simulink model "Maxpid_correction_veleves"  (R2015b)
settings: Solver=ode45  StartTime=0.0  StopTime=1  MaxStep=0.01  RelTol=1e-3
undefined symbols (not defined in the file): Cext, Kd, Ki, Kp
settings Model: Creator=antomart  LastModifiedBy=David
settings DataIOCC: LimitDataPoints=off  SaveFormat=StructureWithTime
settings HardwareCC: ProdWordSize=32  ProdHWDeviceType=Specified
settings ModelReferenceCC: PropagateSignalLabelsOutOfModel=on
settings GRTTargetCC: GeneratePreprocessorConditionals=Disable all

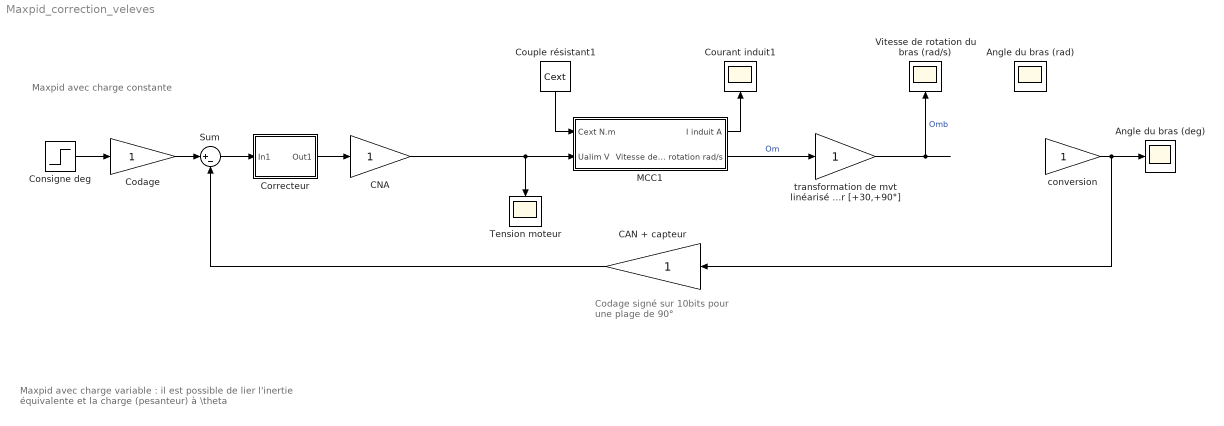
== system Maxpid_correction_veleves ==
  note: Maxpid avec charge variable : il est possible de lier l'inertie équivalente et la charge (pesanteur) à \theta
  note: Maxpid avec charge constante
  note: Codage signé sur 10bits pour une plage de 90°
  Angle du bras (rad) : Scope
  Angle du bras (deg) : Scope
  CAN + capteur : Gain
  CNA : Gain
  Codage : Gain
  Consigne deg : Step  Time=0  After=30  SampleTime=0
  Correcteur : Subsystem
  Couple résistant1 : Constant  Value=Cext
  Courant induit1 : Scope
  MCC1 : Subsystem
  Sum : Sum  Inputs=|+-
  Tension moteur : Scope
  Vitesse de rotation du bras (rad/s) : Scope
  conversion : Gain
  transformation de mvt linéarisé sur [+30,+90°] : Gain
  wires:
  Couple résistant1/1 -> MCC1/1(Cext N.m)
  MCC1/1(I induit A) -> Courant induit1/1
  MCC1/2(Vitesse de rotation rad/s) -> transformation de mvt linéarisé sur [+30,+90°]/1  "Om"
  transformation de mvt linéarisé sur [+30,+90°]/1 -> Vitesse de rotation du bras (rad/s)/1  "Omb"
  ? -> conversion/1, Angle du bras (rad)/1  "Thb (rad)"
  Sum/1 -> Correcteur/1(In1)
  Correcteur/1(Out1) -> CNA/1
  Consigne deg/1 -> Codage/1
  CAN + capteur/1 -> Sum/2
  Codage/1 -> Sum/1
  conversion/1 -> CAN + capteur/1, Angle du bras (deg)/1
  CNA/1 -> MCC1/2(Ualim V), Tension moteur/1

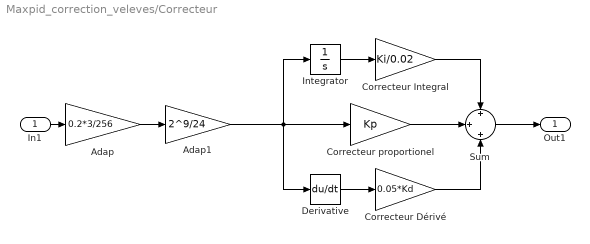
== system Maxpid_correction_veleves/Correcteur ==
  In1 : Inport
  Adap : Gain  Gain=0.2*3/256
  Adap1 : Gain  Gain=2^9/24
  Correcteur Dérivé : Gain  Gain=0.05*Kd
  Correcteur Integral : Gain  Gain=Ki/0.02
  Correcteur proportionel : Gain  Gain=Kp
  Derivative : Derivative
  Integrator : Integrator
  Sum : Sum  Inputs=+|+|+
  Out1 : Outport
  wires:
  In1/1 -> Adap/1
  Integrator/1 -> Correcteur Integral/1
  Correcteur Integral/1 -> Sum/1
  Correcteur proportionel/1 -> Sum/2
  Derivative/1 -> Correcteur Dérivé/1
  Correcteur Dérivé/1 -> Sum/3
  Sum/1 -> Out1/1
  Adap/1 -> Adap1/1
  Adap1/1 -> Derivative/1, Integrator/1, Correcteur proportionel/1

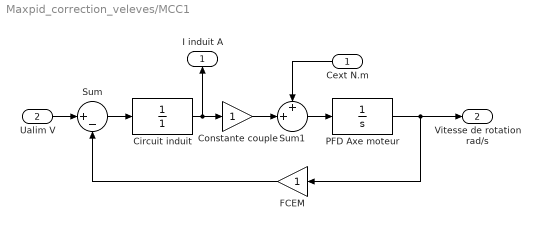
== system Maxpid_correction_veleves/MCC1 ==
  Cext N.m : Inport
  Ualim V : Inport  Port=2
  Circuit induit : TransferFcn  Denominator=[0 1]
  Constante couple : Gain
  FCEM : Gain
  PFD Axe moteur : TransferFcn  Denominator=[1 0]
  Sum : Sum  Inputs=|+-
  Sum1 : Sum  Inputs=++|
  I induit A : Outport
  Vitesse de rotation rad/s : Outport  Port=2
  wires:
  PFD Axe moteur/1 -> Vitesse de rotation rad/s/1, FCEM/1
  Sum1/1 -> PFD Axe moteur/1
  Constante couple/1 -> Sum1/2
  Circuit induit/1 -> Constante couple/1, I induit A/1
  Sum/1 -> Circuit induit/1
  FCEM/1 -> Sum/2
  Cext N.m/1 -> Sum1/1
  Ualim V/1 -> Sum/1
